simulink model "lab2"  (R2019a)
settings: Solver=VariableStepAuto  StartTime=0.0  StopTime=10.0  RelTol=1e-3
settings Model: Creator=T.S  LastModifiedBy=T.S

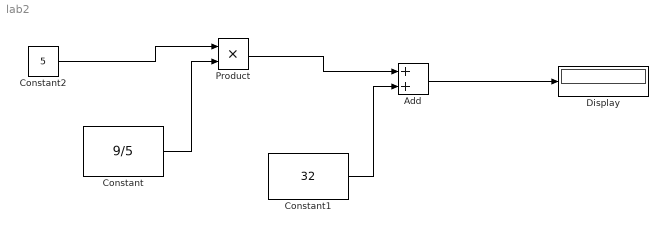
== system lab2 ==
  Add : Sum
  Constant : Constant  Value=9/5
  Constant1 : Constant  Value=32
  Constant2 : Constant  Value=5
  Display : Display
  Product : Product
  wires:
  Constant/1 -> Product/2
  Constant2/1 -> Product/1
  Add/1 -> Display/1
  Constant1/1 -> Add/2
  Product/1 -> Add/1
